simulink model "AUAV_V3_33EP512MU810_SPI_MPU6000__I2C_HMC5883_SensorsTest"  (Simulink 7.5)
settings: Solver=FixedStepDiscrete  StartTime=0.0  StopTime=10.0  FixedStep=0.001  RelTol=1e-3
undefined symbols (not defined in the file or in its folder): A0, A14, A15, A2, A3, A5, A6, B0, D0, D11, D14, D15, D8, F2, F3, F4, F5, G0, G15, IC1max, Max, ms, OC1max, P100, P101, P112, P127, P16, P21, P30, P31, P64, P72, P75, P78, P79, P80, P82, P83, P98, P99, Pin, Resol, Timer, us
libraries: MCHP_Blockset x23, simulink x8
(part 2 of 2)

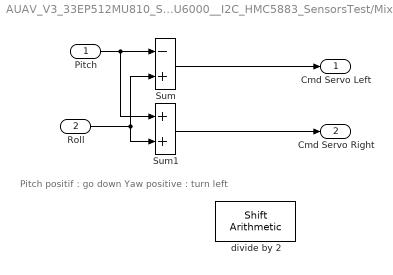
== system AUAV_V3_33EP512MU810_SPI_MPU6000__I2C_HMC5883_SensorsTest/Mixing ==
  note: Pitch positif : go down
      | Yaw positive : turn left
  Pitch : Inport
  Roll : Inport  Port=2
  Sum : Sum  Inputs=-+  SaturateOnIntegerOverflow=on  OutDataTypeStr=Inherit: Same as first input
  Sum1 : Sum  SaturateOnIntegerOverflow=on  OutDataTypeStr=Inherit: Same as first input
  divide by 2 : simulink/Logic and Bit Operations/Shift Arithmetic  SystemSampleTime=-1  nBitShiftRight=1  nBinPtShiftRight=0
  Cmd Servo Left : Outport
  Cmd Servo Right : Outport  Port=2
  wires:
  Pitch/1 -> Sum1/1, Sum/1
  Roll/1 -> Sum/2, Sum1/2
  Sum/1 -> Cmd Servo Left/1
  Sum1/1 -> Cmd Servo Right/1

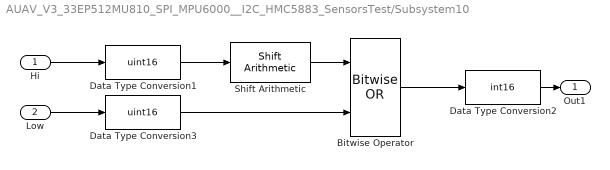
== system AUAV_V3_33EP512MU810_SPI_MPU6000__I2C_HMC5883_SensorsTest/Subsystem10 ==
  Hi : Inport
  Low : Inport  Port=2
  Bitwise Operator : simulink/Logic and Bit Operations/Bitwise Operator  logicop=OR  UseBitMask=off  NumInputPorts=2  BitMask=bin2dec('11011001')  BitMaskRealWorld=Stored Integer
  Data Type Conversion1 : DataTypeConversion  OutDataTypeMode=uint16  OutDataTypeStr=uint16  ConvertRealWorld=Stored Integer (SI)
  Data Type Conversion2 : DataTypeConversion  OutDataTypeMode=int16  OutDataTypeStr=int16  ConvertRealWorld=Stored Integer (SI)
  Data Type Conversion3 : DataTypeConversion  OutDataTypeMode=uint16  OutDataTypeStr=uint16  ConvertRealWorld=Stored Integer (SI)
  Shift Arithmetic : simulink/Logic and Bit Operations/Shift Arithmetic  SystemSampleTime=-1  nBitShiftRight=8  nBinPtShiftRight=0
  Out1 : Outport
  wires:
  Hi/1 -> Data Type Conversion1/1
  Bitwise Operator/1 -> Data Type Conversion2/1
  Data Type Conversion2/1 -> Out1/1
  Data Type Conversion1/1 -> Shift Arithmetic/1
  Shift Arithmetic/1 -> Bitwise Operator/1
  Low/1 -> Data Type Conversion3/1
  Data Type Conversion3/1 -> Bitwise Operator/2

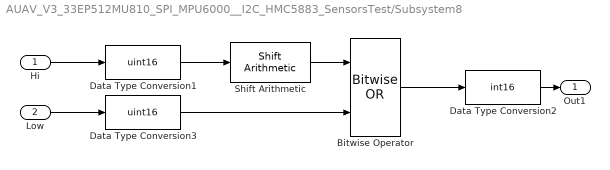
== system AUAV_V3_33EP512MU810_SPI_MPU6000__I2C_HMC5883_SensorsTest/Subsystem8 ==
  Hi : Inport
  Low : Inport  Port=2
  Bitwise Operator : simulink/Logic and Bit Operations/Bitwise Operator  logicop=OR  UseBitMask=off  NumInputPorts=2  BitMask=bin2dec('11011001')  BitMaskRealWorld=Stored Integer
  Data Type Conversion1 : DataTypeConversion  OutDataTypeMode=uint16  OutDataTypeStr=uint16  ConvertRealWorld=Stored Integer (SI)
  Data Type Conversion2 : DataTypeConversion  OutDataTypeMode=int16  OutDataTypeStr=int16  ConvertRealWorld=Stored Integer (SI)
  Data Type Conversion3 : DataTypeConversion  OutDataTypeMode=uint16  OutDataTypeStr=uint16  ConvertRealWorld=Stored Integer (SI)
  Shift Arithmetic : simulink/Logic and Bit Operations/Shift Arithmetic  SystemSampleTime=-1  nBitShiftRight=8  nBinPtShiftRight=0
  Out1 : Outport
  wires:
  Hi/1 -> Data Type Conversion1/1
  Bitwise Operator/1 -> Data Type Conversion2/1
  Data Type Conversion2/1 -> Out1/1
  Data Type Conversion1/1 -> Shift Arithmetic/1
  Shift Arithmetic/1 -> Bitwise Operator/1
  Low/1 -> Data Type Conversion3/1
  Data Type Conversion3/1 -> Bitwise Operator/2

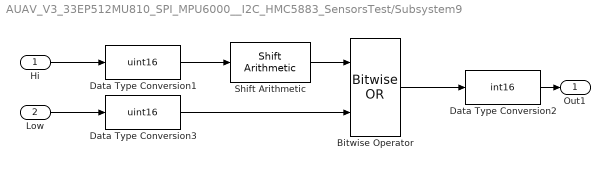
== system AUAV_V3_33EP512MU810_SPI_MPU6000__I2C_HMC5883_SensorsTest/Subsystem9 ==
  Hi : Inport
  Low : Inport  Port=2
  Bitwise Operator : simulink/Logic and Bit Operations/Bitwise Operator  logicop=OR  UseBitMask=off  NumInputPorts=2  BitMask=bin2dec('11011001')  BitMaskRealWorld=Stored Integer
  Data Type Conversion1 : DataTypeConversion  OutDataTypeMode=uint16  OutDataTypeStr=uint16  ConvertRealWorld=Stored Integer (SI)
  Data Type Conversion2 : DataTypeConversion  OutDataTypeMode=int16  OutDataTypeStr=int16  ConvertRealWorld=Stored Integer (SI)
  Data Type Conversion3 : DataTypeConversion  OutDataTypeMode=uint16  OutDataTypeStr=uint16  ConvertRealWorld=Stored Integer (SI)
  Shift Arithmetic : simulink/Logic and Bit Operations/Shift Arithmetic  SystemSampleTime=-1  nBitShiftRight=8  nBinPtShiftRight=0
  Out1 : Outport
  wires:
  Data Type Conversion3/1 -> Bitwise Operator/2
  Low/1 -> Data Type Conversion3/1
  Shift Arithmetic/1 -> Bitwise Operator/1
  Data Type Conversion1/1 -> Shift Arithmetic/1
  Data Type Conversion2/1 -> Out1/1
  Bitwise Operator/1 -> Data Type Conversion2/1
  Hi/1 -> Data Type Conversion1/1
